simulink subsystem "NoBattery"  (R2025a)
settings: Solver=VariableStepAuto  StartTime=0.0  StopTime=10.0  RelTol=1e-3
settings Model: ModifiedByFormat=The MathWorks, Inc.  Creator=The MathWorks, Inc.  LastModifiedBy=The MathWorks, Inc.
settings RTWCC: GPUComputeCapability=3.5

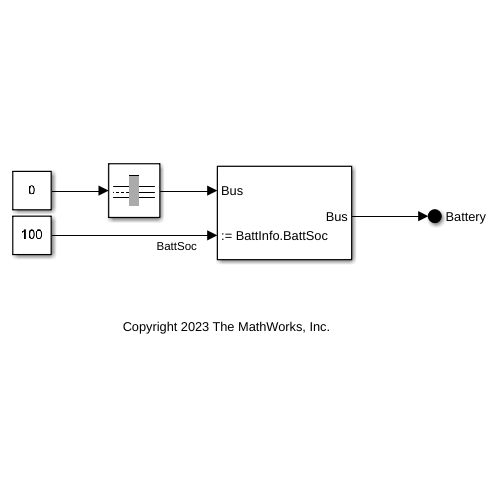
[thumbnail: Simulink's stored preview of the top-level diagram]
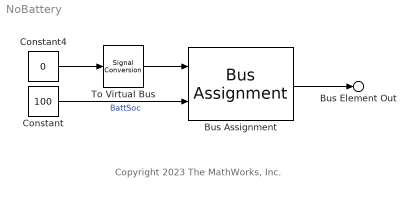
== system NoBattery ==
  note: Copyright 2023 The MathWorks, Inc.
  Bus Assignment : BusAssignment  AssignedSignals=BattInfo.BattSoc
  Constant : Constant  Value=100  SampleTime=-1
  Constant4 : Constant  Value=0  OutDataTypeStr=Bus: BatteryBUS  SampleTime=Inf
  To Virtual Bus : SignalConversion  ConversionOutput=Virtual bus  OverrideOpt=off
  Bus Element Out : Outport  PortName=Battery
  wires:
  To Virtual Bus/1 -> Bus Assignment/1
  Bus Assignment/1 -> Bus Element Out/1
  Constant4/1 -> To Virtual Bus/1
  Constant/1 -> Bus Assignment/2  "BattSoc"
